simulink model "STModel_with_MMAE"  (R2018b)
settings: Solver=FixedStepDiscrete  StartTime=0.0  StopTime=6  FixedStep=Tsmall  RelTol=1e-3  EnableMultiTasking=on
PreLoadFcn:
  | if exist('tl_preloadfcn','file'), tl_preloadfcn(gcs,403); end
PostLoadFcn:
  | if exist('tl_postloadfcn','file'), tl_postloadfcn(gcs,403); end
InitFcn:
  | if exist('tlds_init','file'), tlds_init(gcs); end
StartFcn:
  | if exist('tlds_start','file'), tlds_start(gcs); end
StopFcn:
  | if exist('tlds_stop','file'), tlds_stop(gcs); end
values from neighbouring files (symbols this model uses):
  l = obj.vehicleParameters.l_r + obj.vehicleParameters.l_f    [SimplifiedKinematicBicycleModel.m]
  l_r = obj.vehicleParameters.l_r    [KinematicBicycleModel.m]
  Ts = 0.1    [KinematicBicycleModel.m]    (also in LeftLaneChangeSinusoidalMotionModel.m; LinearizedBicycleModel.m; SimplifiedKinematicBicycleModel.m; amm_rel_test.m)
  Ts_bp = 0.01    [initialization.m]    (also in laneChangeSinusoidalFcn.m; laneChangeSinusoidalJacobianFcn.m; leftLaneChangeParametricFcn.m; leftLaneChangeParametricWithAccFcn.m)
  vx = X(2)    [cv_model_fun.m]    (also in initialization.m = 10)
  vy = X(4)    [cv_model_fun.m]    (also in initialization.m = 0)
  x = X(1)    [KinematicBicycleModel.m]    (also in SimplifiedKinematicBicycleModel.m; behavior_model.m = 0:0.01:20; cca_model_fun.m; ctra_model_fun.m)
  y = X(2)    [KinematicBicycleModel.m]    (also in SimplifiedKinematicBicycleModel.m; behavior_model.m = [distances velocities]; cca_model_fun.m; ctra_model_fun.m)
undefined symbols (not defined in the file or in its folder): alpha_f0, alpha_r0, Bm1, Bsc, Bx_ash_f, Bx_ash_r, Bx_snow_f, Bx_snow_r, Bx_wash_f, Bx_wash_r, By_ash_f, By_ash_r, By_snow_f, By_snow_r, By_wash_f, By_wash_r, Cx_ash_f, Cx_ash_r, Cx_snow_f, Cx_snow_r, Cx_wash_f, Cx_wash_r, Cy_ash_f, Cy_ash_r, Cy_snow_f, Cy_snow_r, Cy_wash_f, Cy_wash_r, Ex_ash_f, Ex_ash_r, Ex_snow_f, Ex_snow_r, Ex_wash_f, Ex_wash_r, Ey_ash_f, Ey_ash_r, Ey_snow_f, Ey_snow_r, Ey_wash_f, Ey_wash_r, g, Im1, Isw, Iw, Iz, Kb1, Ks1, kt1, l_f, m, mu_x_ash_f, mu_x_ash_r, mu_x_snow_f, mu_x_snow_r, mu_x_wash_f, mu_x_wash_r, mu_y_ash_f, mu_y_ash_r, mu_y_snow_f, mu_y_snow_r ... (+18)
libraries: simulink x6
(part 2 of 2)

== matlab function STModel_with_MMAE/Behavior Identification/KF for straight/MATLAB Function ==
  data: X input; P input; u input; X_hat_plus output; y_tilde input; P_plus output; ek_minus output; ek_m_covariance output; wk output; wk_prev input; p_yk_xkminus output; K output
function [X_hat_plus, P_plus, ek_minus, ek_m_covariance, wk, p_yk_xkminus, K] = kalmanFilterCustom(X, P, u, y_tilde, wk_prev)

    %%
    %TODO: See how can this be moved out of the function later
    %sampling time
    Ts_bp = 0.01;

    % measurement noise covariance
%     R = [0.2 0; 0 0.2];
    R = [0.025 0; 0 0.025];
    
    % process noise covariance
%     Q = diag([0.5 5.0 0.5 5.0]);
    Q = diag([0.005 0.005 0.005 0.005]);

    % states - X = [x vx y vy] - 
    
    Ak = [1 Ts_bp 0 0; 0 1 0 0; 0 0 1 Ts_bp; 0 0 0 1];
    Bk = 0;
    Ck = [1 0 0 0; 0 0 1 0];
    Dk = 0;

    %%
    % Now estimate states using kalman filter
    
    %predict
    xhat_minus = Ak * X + Bk * u;
    P_minus = (Ak * P *Ak') + Ts_bp*Q;
    yhat_minus = Ck * xhat_minus;

    %correct
    ek_minus = y_tilde - yhat_minus;    %residual
    ek_m_covariance = Ck * P_minus *Ck' + R;    %residual covariance
    K = P_minus * Ck' * inv(ek_m_covariance);
    X_hat_plus = xhat_minus + K * ek_minus;
    P_plus = (eye(4) - K * Ck) * P_minus;
    
    %calculate MMAE weights
    p_yk_xkminus = 1/sqrt(det(2*pi*ek_m_covariance))*exp(-1/2 * ek_minus'* inv(ek_m_covariance) * ek_minus);
    wk = wk_prev * p_yk_xkminus;
    
    %This will be likely outside
    %e = xhat_plus - x(:, i+1);
    
end

== matlab function STModel_with_MMAE/Behavior Identification/EKF for Left Lane Change/MATLAB Function2 ==
  data: X input; P input; u input; X_hat_plus output; y_tilde input; P_plus output; ek_minus output; ek_m_covariance output; wk output; p_yk_xkminus output; wk_prev input; maneuver_length input
function [X_hat_plus, P_plus, ek_minus, ek_m_covariance, wk, p_yk_xkminus] = EKFLeftLaneChangeCustom(X, P, u, y_tilde, wk_prev, maneuver_length)

    %%
    %TODO: See how can this be moved out of the function later
    %sampling time
    Ts_bp = 0.01;
%     maneuver_length = 150;  %m
    lane_center_to_center_distance = 3.5;   %meters

    % measurement noise covariance
%     R = [0.2 0; 0 0.2];
    R = [0.025 0; 0 0.025];
    
    % process noise covariance
%     Q = diag([0.5 5.0 0.5 5.0]);
    Q = diag([0.005 0.005 0.005 0.005]);

    % states - X = [x vx y vy] -     
    Ck = [1 0 0 0; 0 0 1 0];

    F = leftLaneChangeParametricJacobianFcn(X, u, maneuver_length, lane_center_to_center_distance);
    %%
    % Now estimate states using kalman filter
    
    %predict
    xhat_minus = leftLaneChangeParametricFcn(X, u, maneuver_length, lane_center_to_center_distance);
    P_minus = (F * P * F') + Ts_bp*Q;
    yhat_minus = Ck * xhat_minus;

    %correct
    ek_minus = y_tilde - yhat_minus;    %residual
    ek_m_covariance = Ck * P_minus *Ck' + R;    %residual covariance
    K = P_minus * Ck' * inv(ek_m_covariance);
    X_hat_plus = xhat_minus + K * ek_minus;
    P_plus = (eye(4) - K * Ck) * P_minus;
    
    %calculate MMAE weights
    p_yk_xkminus = 1/sqrt(det(2*pi*ek_m_covariance))*exp(-1/2 * ek_minus'* inv(ek_m_covariance) * ek_minus);
    wk = wk_prev * p_yk_xkminus;

    
end
